simulink subsystem "consensusADMM"  (R2023b)
settings: Solver=VariableStepAuto  StartTime=0.0  StopTime=10.0  RelTol=1e-3
undefined symbols (not defined in the file): c
settings Model: Creator=is123  LastModifiedBy=is123
settings OptimizationCC: ReuseModelBlockBuffer=off

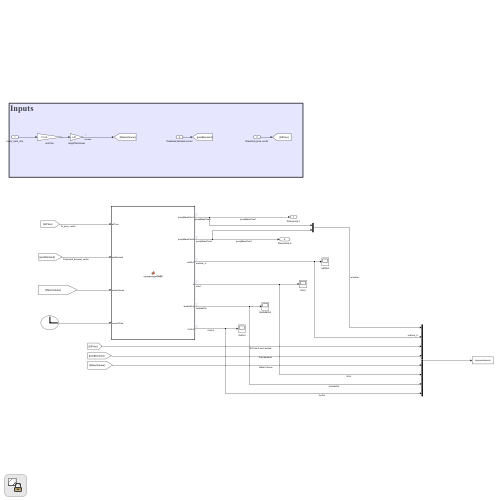
[thumbnail: Simulink's stored preview of the top-level diagram]
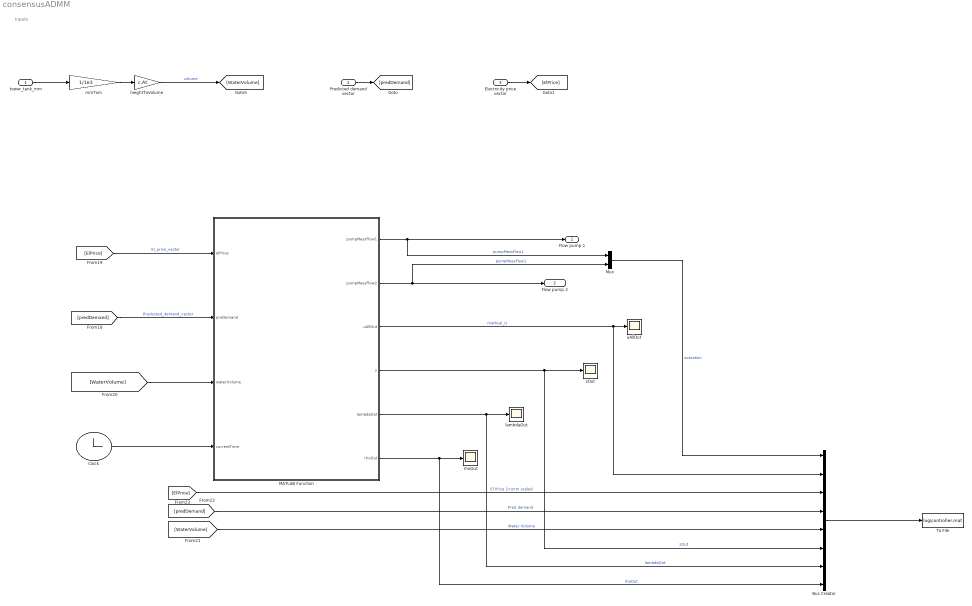
== system consensusADMM ==
  note: Inputs
  tower_tank_mm : Inport
  Predicted demand vector : Inport  Port=2
  Electricity price vector : Inport  Port=3
  Bus Creator : BusCreator  Inputs=8
  Clock : Clock
  MATLAB Function : MATLAB Function  TreatAsAtomicUnit=on  SystemSampleTime=600
  Mux : Mux  Inputs=2
  To File : ToFile  Filename=log\controller.mat  MatrixName=ctrl  SaveFormat=Timeseries
  heightToVolume : Gain  Gain=c.At
  lambdaOut : Scope
  mmTom : Gain  Gain=1/1e3
  rhoOut : Scope
  uAllOut : Scope
  zOut : Scope
  Flow pump 1 : Outport
  Flow pump 2 : Outport  Port=2
  wires:
  mmTom/1 -> heightToVolume/1
  tower_tank_mm/1 -> mmTom/1
  Predicted demand vector/1 -> [predDemand]
  Electricity price vector/1 -> [ElPrice]
  [WaterVolume] -> MATLAB Function/3(waterVolume)
  MATLAB Function/2(pumpMassFlow2) -> Flow pump 2/1, Mux/2  "pumpMassFlow1"
  MATLAB Function/1(pumpMassFlow1) -> Flow pump 1/1, Mux/1  "pumpMassFlow1"
  MATLAB Function/4(z) -> zOut/1, Bus Creator/6  "zOut"
  MATLAB Function/5(lambdaOut) -> lambdaOut/1, Bus Creator/7  "lambdaOut"
  Bus Creator/1 -> To File/1
  heightToVolume/1 -> [WaterVolume]  "volume"
  [predDemand] -> MATLAB Function/2(preDemand)  "Preducted_demand_vector"
  [ElPrice] -> MATLAB Function/1(elPrice)  "El_price_vector"
  MATLAB Function/3(uAllOut) -> uAllOut/1, Bus Creator/2  "mathcal_U"
  Mux/1 -> Bus Creator/1  "actuation"
  Clock/1 -> MATLAB Function/4(currentTime)
  MATLAB Function/6(rhoOut) -> Bus Creator/8, rhoOut/1  "rhoOut"
  [WaterVolume] -> Bus Creator/5  "Water Volume"
  [predDemand] -> Bus Creator/4  "Pred demand"
  [ElPrice] -> Bus Creator/3  "El Price 2-norm scaled"

== matlab function consensusADMM/MATLAB Function ==
  data: elPrice input; pumpMassFlow1 output; preDemand input; waterVolume input; pumpMassFlow2 output; uAllOut output; z output; lambdaOut output; currentTime input; rhoOut output
function [pumpMassFlow1, pumpMassFlow2, uAllOut,z,lambdaOut,rhoOut] = consensusADMM(elPrice,preDemand,waterVolume,currentTime)
    %It is desired to keep the old solution for the inputs and z to inital
    %the next optimization problem, likewise it is desired to use the
    %peanlty parameter rho from the previous problem. To obtain this the
    %following is needed
     coder.extrinsic("pump1Casadi") 
     coder.extrinsic("pump2Casadi")
     coder.extrinsic("WaterTowerCasadi")
    persistent z1 uAll rho rhoSave
        %Getting scaled standard constants to set the inital values 
      c=scaled_standard_constants;  
    if isempty(z1) || isempty(uAll) ||isempty(rho) || isempty(rhoSave)
        z1=zeros(c.Nu*c.Nc,1);
        uAll=zeros(c.Nu*c.Nc,c.Nu+1);
        rho=c.rho; 
        rhoSave=c.rho;
    end

  %setting some of the inputs, because Simulink wants it
  xBar=zeros(c.Nu*c.Nc,c.varying_rho_iterations_numbers); 
  rhoOut=rho; 

    % Scaling the eletricity price if it is desired: 
    if c.scaledEletricityPrice == true
        elPrice=elPrice/norm(elPrice); 
    end 
  


%Giving the system 10 minuts to start up! setting the output to zero in these cases      
if currentTime < 200
        z=zeros(c.Nu*c.Nc,1);
        uAllOut=zeros(c.Nu*c.Nc,c.Nu+1);
        pumpMassFlow1=0; 
        pumpMassFlow2=0; 
        lambdaOut = zeros(c.Nc*c.Nu,c.Nu+1); 
else 
    
    % Updating inital geuss for consensus ADMM 
    x=zeros(c.Nc*c.Nu,c.Nu+1);
    x(:,1)=[uAll(c.Nu+1:end,1);uAll(end-c.Nu+1:end,1)]; 
    x(:,2)=[uAll(c.Nu+1:end,2);uAll(end-c.Nu+1:end,2)]; 
    x(:,3)=[uAll(c.Nu+1:end,3);uAll(end-c.Nu+1:end,3)];
    z=[z1(c.Nu+1:end,1);z1(end-c.Nu+1:end,1)];
    
    %Setting a few needed matrixes to zero: 
    lambdaTilde=zeros(c.Nc*c.Nu,c.Nu+1); 
    lambda = zeros(c.Nc*c.Nu,c.Nu+1); 
    secretScaled=zeros(c.Nc*c.Nu,c.Nu+1); 
    
    yOut=zeros(c.Nu+1,c.Nc*c.Nu,c.Nu+1);
    yOutSum=zeros(c.Nc*c.Nu,1);
    
    %Saving demand and eletricty price in struct 
    data.Je=elPrice; 
    data.d=preDemand; 
    data.V=waterVolume; 

    
    
    %Setting up the matrixes needed for the optimization problem 
    %Summing the two flows for each timestamp in the prediction horzion
    data.A_1=zeros(c.Nc,c.Nu*c.Nc);
    index=1; 
    for i=1:c.Nc
        data.A_1(i,index:index+c.Nu-1) = 1;
        index=index+c.Nu;
    end
    
    %Lower trangiular matrix to add consumption and flows 
    data.A_2 = tril(ones(c.Nc,c.Nc));
    
    
    %Making vi vectors utilized to pick out 1 of the 2 pumps values, add them up
    %used to make extration limit. 
    data.v1=ones(c.Nu*c.Nc,1);
    data.v1(2:2:end) =0; 
    
    data.v2=ones(c.Nu*c.Nc,1);
    data.v2(1:2:end) =0;
    
    %Making matrix which picks out 1 of the pumps for the enitre control
    %horizion
    
    data.A_31=zeros(c.Nc,c.Nu*c.Nc);
    index=1; 
    for i=1:c.Nc
        data.A_31(i,index) = 1;
        index=index+c.Nu;
    end
    
    data.A_32=zeros(c.Nc,c.Nu*c.Nc);
    index=2; 
    for i=1:c.Nc
        data.A_32(i,index) = 1;
        index=index+c.Nu;
    end

    
    tic 
    %% Going though the iterations for consensus ADMM: 
    for k=1:c.iteration
        if c.changeRhoEnd==true
            if k== 1 
                rho=rhoSave; 
            end
        end 
        %Solving the distrubted optimization problem: 
        % x(:,1)=pump1(lambda(:,1),data,z,x(:,1),rho); 
        % x(:,2)=pump2(lambda(:,2),data,z,x(:,2),rho);
        % x(:,3)=WaterTower(lambda(:,3),data,z,x(:,3),rho);
        x(:,1)=pump1Casadi(lambda(:,1),data,z,x(:,1),rho); 
        x(:,2)=pump2Casadi(lambda(:,2),data,z,x(:,2),rho);
        x(:,3)=WaterTowerCasadi(lambda(:,3),data,z,x(:,3),rho);
        %Next it is desired to update the consensus parameter Z, this can
        %be done with or without SMPC
        if c.UseSMPC==true
            %Determine the z part for each of the pumps and making the function
            %output (making it a secret) 
            for index=1:c.Nu+1
                secretScaled(:,index)=c.scaling*(1/(c.Nu+1)*(x(:,index)+1/rho*lambda(:,index))+c.sMPCOffset);
                yOut(:,:,index)=generatedOutFromFunction(secretScaled(:,index));
            end 
            
            % Making the sum 
            yOutSum=yOut(:,:,1)+yOut(:,:,2)+yOut(:,:,3); 
            %Rounding: 
            yOutSum=round(yOutSum); 
            %Getting the secret
            secret=GetFunctionParameter(yOutSum);
        
            % Descaling the secret
            zTilde=(secret)/c.scaling-((c.Nu+1)*c.sMPCOffset);
        else
        %Updating z/updating consensus parameter 
        zTilde = sum(x,2)/(c.Nu+1) + 1/(rho*(c.Nu+1))*sum(lambda,2);
        end
        z = z - 1/(c.Nu+1+1)*(z-zTilde);
        %Updating lambda
        for i=1:c.Nu+1
            lambdaTilde(:,i) = lambda(:,i) + rho*(x(:,i)-z);
        end
            lambda = lambda - 1/(c.Nu+1+1)*(lambda - lambdaTilde);
        
        %If rho should by varyed: 
        if c.varying_rho==true && k<c.varying_rho_iterations_numbers+1 
            %% Setting primal and dual residal to zero: 
            r=0;
            s=0; 
            %% Determine xBar, this can be done secure using sMPC or just the normal way:
            if c.UseSMPC==true

                %Determining the value out of the function 
                for index=1:c.Nu+1
                    secretScaled(:,index)=c.scaling*((x(:,1)/(c.Nu+1))+c.sMPCOffset);
                    yOut(:,:,index)=generatedOutFromFunction(secretScaled(:,index));
                end 
                
                % Making the sum 
                yOutSum=yOut(:,:,1)+yOut(:,:,2)+yOut(:,:,3); 
                %Making rounding: 
                yOutSum=round(yOutSum); 
                %Getting the secret
                secret=GetFunctionParameter(yOutSum);
                %Determine xBar:
                xBar(:,k)=(secret)/c.scaling-((c.Nu+1)*c.sMPCOffset)
            else 
                xBar(:,k)=sum(x,2)/(c.Nu+1)
            end 
            %% Determining the primal residual this  can be done secure by secure by using SMPC
                
            if c.UseSMPC==true
                %Determining the value out of the function 
                for index=1:c.Nu+1
                    secretScaled(:,index)=c.scaling*(norm(x(:,index)-xBar(:,k))^2);
                    yOut(:,:,index)=generatedOutFromFunction(secretScaled(:,index));
                end 
                
                % Making the sum 
                yOutSum=yOut(:,:,1)+yOut(:,:,2)+yOut(:,:,3); 
                %Making rounding: 
                yOutSum=round(yOutSum); 

                %Determining the secret: 
                secret=GetFunctionParameter(yOutSum);
                %Determing the primal residual
                r=secret/c.scaling; 
                r=sqrt(r); 
            else 
                %Determining primal residual 

                 for index=1:c.Nu+1 
                    r=norm(x(:,index)-xBar(:,k))^2+r
                 end 
                 r=sqrt(r);
            end 
                %Determining dual residual 
                if k==1
                    s=sqrt((c.Nu+1)*rho^2*norm(xBar(:,k))^2)
                else
                    s=sqrt((c.Nu+1)*rho^2*norm(xBar(:,k)-xBar(:,k-1))^2)
                end 
                %Determine if the value of rho should change 
                 if r >c.mu*s 
                    rho=c.tauIncr*rho; 
                 elseif s>c.mu*r 
                     rho=rho/c.tauDecr; 
                 end 
                  
                 rhoSave=rho; 
        end  
        if c.changeRhoEnd==true
            if k >=c.iterationRhoChange 
                rho=c.RhoEnd;
            end
        end 
        rho
    end %End for loop for iterations
    %Determinging the time it took
    
    %Setting the output of the function 
    pumpMassFlow1=x(1,1);
    pumpMassFlow2=x(2,2);
        uAllOut=x; 
        rhoOut=rho; 
    lambdaOut=lambda; 
end %End if statement
    
    

    

end %end function
